simulink model "Discrete_Bicycle_Simulink_Model"  (R2024a)
settings: Solver=ode4  StartTime=0.0  StopTime=10  FixedStep=0.01  RelTol=1e-3
values from neighbouring files (symbols this model uses):
  Ad = sysd.A    [Discrete_SS_with_Discrete_LQG.m]
  Aobs = Ad - Ld*Cd    [Discrete_SS_with_Discrete_LQG.m]
  Bd = sysd.B    [Discrete_SS_with_Discrete_LQG.m]
  Bobs = [Ld, Bd]    [Discrete_SS_with_Discrete_LQG.m]
  c = 0.08    [Discrete_SS_with_Discrete_LQG.m]
  Cd = sysd.C    [Discrete_SS_with_Discrete_LQG.m]
  Cobs = eye(4)    [Discrete_SS_with_Discrete_LQG.m]
  Dd = sysd.D    [Discrete_SS_with_Discrete_LQG.m]
  Dobs = zeros(4, size(Bobs,2))    [Discrete_SS_with_Discrete_LQG.m]
  Kd = dlqr(Ad, Bd, Q, R)    [Discrete_SS_with_Discrete_LQG.m]
  lambda = pi/10    (= 0.314159265359)    [Discrete_SS_with_Discrete_LQG.m]
  Ts = 0.01    [Discrete_SS_with_Discrete_LQG.m]
  v = 15    [Discrete_SS_with_Discrete_LQG.m]
  w = 1.02    [Discrete_SS_with_Discrete_LQG.m]
  x0 = [0.2 ;0 ;1.5 ;0]    [Discrete_SS_with_Discrete_LQG.m]
  xhat0 = [0. ;0 ;0 ;0]    [Discrete_SS_with_Discrete_LQG.m]
undefined symbols (not defined in the file or in its folder): DiscIntNeverNeededParam
settings Model: Creator=Vipuls  LastModifiedBy=Vipuls

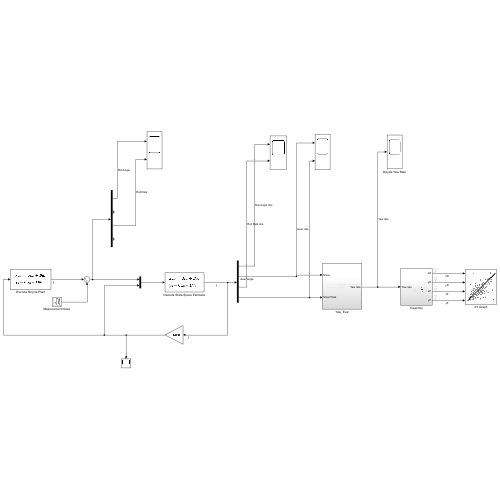
[thumbnail: Simulink's stored preview of the top-level diagram]
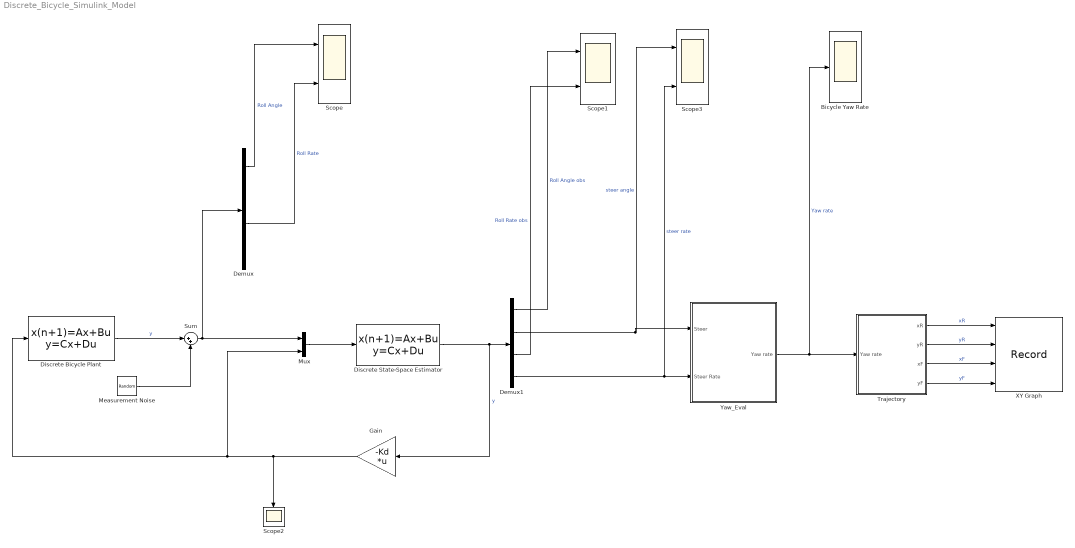
== system Discrete_Bicycle_Simulink_Model ==
  Bicycle Yaw Rate : Scope
  Demux : Demux
  Demux1 : Demux
  Discrete Bicycle Plant : DiscreteStateSpace  A=Ad  B=Bd  C=Cd  D=Dd  InitialCondition=x0  SampleTime=Ts
  Discrete State-Space Estimator : DiscreteStateSpace  A=Aobs  B=Bobs  C=Cobs  D=Dobs  InitialCondition=xhat0  SampleTime=-1
  Gain : Gain  Gain=-Kd  Multiplication=Matrix(K*u)
  Measurement Noise : RandomNumber  Variance=[0.0001, 0.0001, 0.0001, 0.0001]  SampleTime=Ts
  Mux : Mux  Inputs=2
  Scope : Scope  NumInputPorts=2
  Scope1 : Scope  NumInputPorts=2
  Scope2 : Scope
  Scope3 : Scope  NumInputPorts=2
  Sum : Sum  Inputs=|++
  Trajectory : Subsystem
  XY Graph : Record  FileSettingsInternal="{\"entries\":[{\"content\":{\"excelSettings\":{\"content\":{},\"type\":\"Streamout.ExcelSettings\"}},\"type\":\"Streamout.FileSettingStorage\",\"uuid\":\"\"}],\"packageUris\":[\"http:\\/\\/schema.mathworks.com\\/mf0\\/streamout_blocks\\/R2020a\"],\"version\":\"1.0\"}"  Layout=[1 1]  SignalsInternal="{\"entries\":[{\"content\":{\"signals\":[{\"content\":{\"blockPath\":[],\"dimensions\":[1],\"domain\":\"\",\"lineColor\":\"#fe330a\",\"lineWidth\":2,\"port\":1,\"sid\":[\"\"],\"signalID\":1,\"signalName\":\"xR\"},\"type\":\"RecordBlkView.Signal\",\"uuid\":\"\"},{\"content\":{\"blockPath\":[],\"dimensions\":[1],\"domain\":\"\",\"lineColor\":\"#22b573\",\"lineWidth\":2,\"port\":2,\"sid\":[\"\"],\"signalID\":2,\"signalName\":\"yR\"},\"type\":\"RecordBlkView.Signal\",\"uuid\":\"\"},{\"content\":{\"blockPath\":[],\"dimensions\":[1],\"domain\":\"\",\"lineColor\":\"#0072bd\",\"lineWidth\":2,\"port\":3,\"sid\":[\"\"],\"signalID\":3,\"signalName\":\"xF\"},\"type\":\"RecordBlkView.Signal\",\"uuid\":\"\"},{\"content\":{\"blockPath\":[],\"dimensions\":[1],\"domain\":\"\",\"lineColor\":\"#d95319\",\"lineWidth\":2,\"port\":4,\"sid\":[\"\"],\"signalID\":4,\"signalName\":\"yF\"},\"type\":\"RecordBlkView.Signal\",\"uuid\":\"\"}]},\"type\":\"RecordBlkView.InputSignals\",\"uuid\":\"\"}],\"packageUris\":[\"http:\\/\\/schema.mathworks.com\\/mf0\\/streamout_blocks\\/R2020a\"],\"version\":\"1.0\"}"  VisualizationBindings="{\"xyplotplugin\":{\"info\":[{\"series\":[],\"subplotID\":1}]}}"  CompatibilityTag=XY
  Yaw_Eval : Subsystem
  wires:
  Measurement Noise/1 -> Sum/2
  Sum/1 -> Mux/1, Demux/1
  Mux/1 -> Discrete State-Space Estimator/1
  Gain/1 -> Discrete Bicycle Plant/1, Mux/2, Scope2/1
  Demux/1 -> Scope/1  "Roll Angle"
  Demux/3 -> Scope/2  "Roll Rate"
  Discrete State-Space Estimator/1 -> Gain/1, Demux1/1  "y"
  Demux1/3 -> Scope1/2  "Roll Rate obs"
  Demux1/1 -> Scope1/1  "Roll Angle obs"
  Discrete Bicycle Plant/1 -> Sum/1  "y"
  Demux1/4 -> Scope3/2, Yaw_Eval/2(Steer Rate)  "steer rate"
  Demux1/2 -> Yaw_Eval/1(Steer), Scope3/1  "steer angle"
  Yaw_Eval/1(Yaw rate) -> Bicycle Yaw Rate/1, Trajectory/1(Yaw rate)  "Yaw rate"
  Trajectory/1(xR) -> XY Graph/1  "xR"
  Trajectory/2(yR) -> XY Graph/2  "yR"
  Trajectory/3(xF) -> XY Graph/3  "xF"
  Trajectory/4(yF) -> XY Graph/4  "yF"

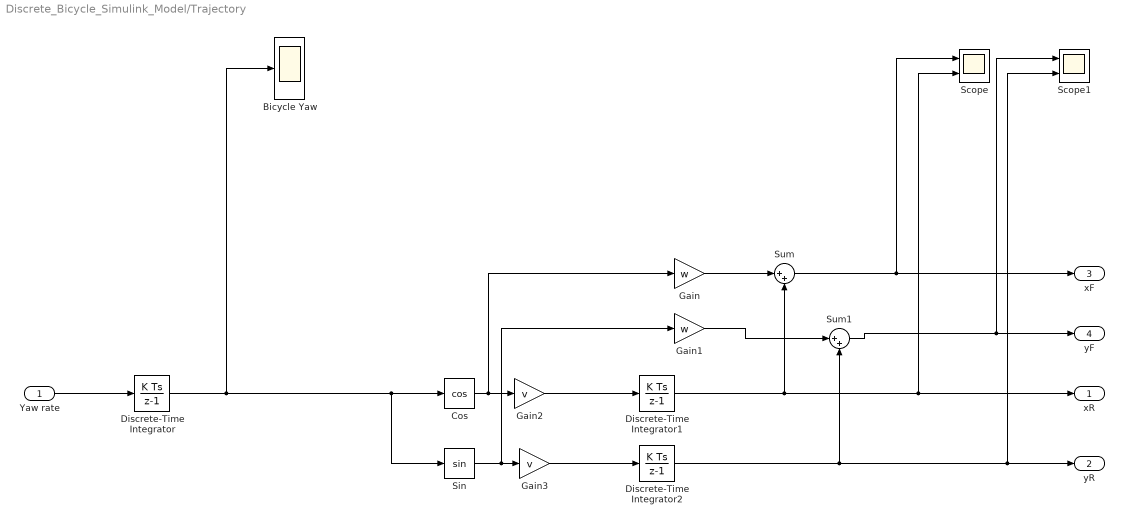
== system Discrete_Bicycle_Simulink_Model/Trajectory ==
  Yaw rate : Inport
  Bicycle Yaw : Scope
  Cos : Trigonometry  Operator=cos
  Discrete-Time Integrator : DiscreteIntegrator  SampleTime=Ts  ICPrevOutput=DiscIntNeverNeededParam  ICPrevScaledInput=DiscIntNeverNeededParam
  Discrete-Time Integrator1 : DiscreteIntegrator  SampleTime=Ts  ICPrevOutput=DiscIntNeverNeededParam  ICPrevScaledInput=DiscIntNeverNeededParam
  Discrete-Time Integrator2 : DiscreteIntegrator  SampleTime=Ts  ICPrevOutput=DiscIntNeverNeededParam  ICPrevScaledInput=DiscIntNeverNeededParam
  Gain : Gain  Gain=w
  Gain1 : Gain  Gain=w
  Gain2 : Gain  Gain=v
  Gain3 : Gain  Gain=v
  Scope : Scope  NumInputPorts=2
  Scope1 : Scope  NumInputPorts=2
  Sin : Trigonometry
  Sum : Sum  Inputs=|++
  Sum1 : Sum  Inputs=|++
  xR : Outport
  yR : Outport  Port=2
  xF : Outport  Port=3
  yF : Outport  Port=4
  wires:
  Cos/1 -> Gain/1, Gain2/1
  Gain3/1 -> Discrete-Time Integrator2/1
  Gain2/1 -> Discrete-Time Integrator1/1
  Discrete-Time Integrator1/1 -> Scope/2, xR/1, Sum/2
  Discrete-Time Integrator2/1 -> Sum1/2, Scope1/2, yR/1
  Yaw rate/1 -> Discrete-Time Integrator/1
  Discrete-Time Integrator/1 -> Bicycle Yaw/1, Sin/1, Cos/1
  Sin/1 -> Gain1/1, Gain3/1
  Gain1/1 -> Sum1/1
  Gain/1 -> Sum/1
  Sum/1 -> Scope/1, xF/1
  Sum1/1 -> Scope1/1, yF/1

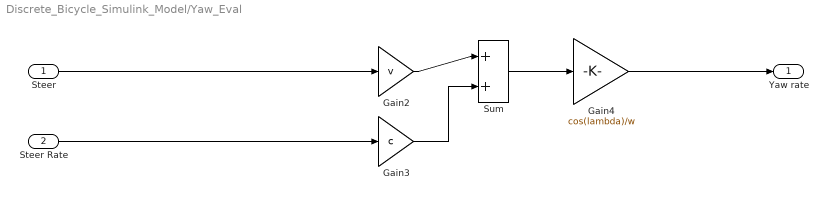
== system Discrete_Bicycle_Simulink_Model/Yaw_Eval ==
  Steer : Inport
  Steer Rate : Inport  Port=2
  Gain2 : Gain  Gain=v
  Gain3 : Gain  Gain=c
  Gain4 : Gain  Gain=cos(lambda)/w
  Sum : Sum  Inputs=|++
  Yaw rate : Outport
  wires:
  Sum/1 -> Gain4/1
  Gain4/1 -> Yaw rate/1
  Gain3/1 -> Sum/2
  Steer Rate/1 -> Gain3/1
  Gain2/1 -> Sum/1
  Steer/1 -> Gain2/1
